simulink library "roblocks"  (Simulink 4.00)
values from neighbouring files (symbols this model uses):
  q = u(1:n)    [sldyn.m]
  qd = u(n+1:2*n)    [sldyn.m]
  qdd = accel(robot, u(1:n), u(n+1:2*n), u(2*n+1:3*n))    [sldyn.m]
undefined symbols (not defined in the file or in its folder): eul2tr, fkine, jacob0, jacobn, rne, robot, rpy2tr, tr2diff, tr2eul, tr2rpy, transl
libraries: simulink3 x2
settings Model: Creator=pic  LastModifiedBy=pic

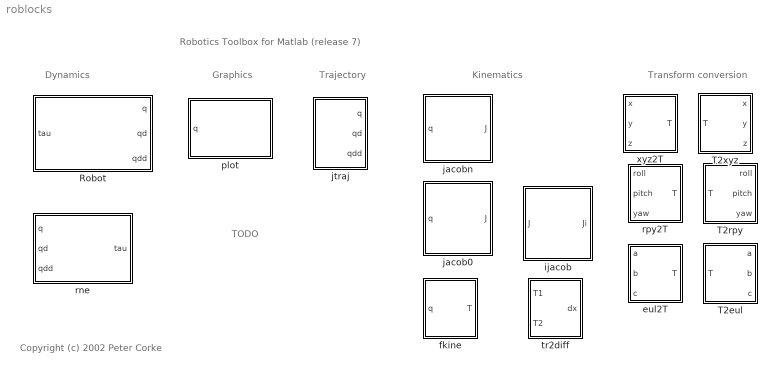
== system roblocks ==
  note: Robotics Toolbox for Matlab (release 7)
  note: TODO
  note: Copyright (c) 2002 Peter Corke
  note: Dynamics
  note: Graphics
  note: Kinematics
  note: Transform conversion
  note: Trajectory
  Robot : Subsystem  mask{robot=robot, q0=[0 0 0 0 0 0]}
      mask prompts: robot "Robot object"; q0 "Initial state"
      mask help: Rigid-body dynamic model of robot.
      mask init:
      | n = robot.n;
      | name = robot.name;
      settings: RTWFcnNameOpts=Auto  RTWFileNameOpts=Auto
      mask Help: Simulates the forward (direct) rigid-body dynamics of the robot described by the given robot object.
      mask Display:
      | port_label('input', 1, 'tau')
      | port_label('output', 1, 'q')
      | port_label('output', 2, 'qd')
      | port_label('output', 3, 'qdd')
      | text(0.1, 0.9,  robot.name, 'horizontalAlignment', 'left')
  T2eul : Subsystem
      settings: RTWFcnNameOpts=Auto  RTWFileNameOpts=Auto
      mask Description: Convert transform to Euler angles.
  T2rpy : Subsystem
      settings: RTWFcnNameOpts=Auto  RTWFileNameOpts=Auto
      mask Description: Convert transform to roll/pitch/yaw angles.
  T2xyz : Subsystem
      settings: RTWFcnNameOpts=Auto  RTWFileNameOpts=Auto
      mask Description: Convert transform to xyz scalars
  eul2T : Subsystem
      settings: RTWFcnNameOpts=Auto  RTWFileNameOpts=Auto
      mask Description: Convert Euler angles to transform.
  fkine : Subsystem  mask{robot=robot}
      mask prompts: robot "Robot object"
      mask help: Robot forward kinematics.
      settings: RTWFcnNameOpts=Auto  RTWFileNameOpts=Auto
      mask Help: Compute homogeneous transform for robot end-effector given joint angles.
      mask Display:
      | port_label('input', 1, 'q')
      | port_label('output', 1, 'T')
      | text(0.9, 0.9, robot.name,  'horizontalAlignment', 'right')
  ijacob : Subsystem
      settings: RTWFcnNameOpts=Auto  RTWFileNameOpts=Auto
      mask Description:
      | Robot inverse Jacobian for world coordinates.
      | 
      | Only valid for square jacobians (ie/ 6DOF robots)
      mask Display:
      | text(0.4, 0.7, 'J', 'verticalAlignment', 'top', 'horizontalAlignment', 'left')
      | text(0.65, 0.65, '-1', 'verticalAlignment', 'bottom', 'horizontalAlignment', 'right')
      | port_label('input', 1, 'J');
      | port_label('output', 1, 'Ji')
  "jacob0 " : Subsystem  mask{robot=robot}
      mask prompts: robot "Robot object"
      mask help: Robot Jacobian for end-effector coordinates
      mask init:
      | n=robot.n;
      settings: RTWFcnNameOpts=Auto  RTWFileNameOpts=Auto
      mask Display:
      | text(0.4, 0.7, 'J', 'verticalAlignment', 'top', 'horizontalAlignment', 'left')
      | text(0.4, 0.7, '0', 'verticalAlignment', 'bottom', 'horizontalAlignment', 'right')
      | text(0.5, 0.2, robot.name,  'horizontalAlignment', 'center')
      | port_label('input', 1, 'q')
      | port_label('output', 1, 'J')
  jacobn : Subsystem  mask{robot=robot}
      mask prompts: robot "Robot object"
      mask help: Robot Jacobian for end-effector coordinates
      mask init:
      | n=robot.n;
      settings: RTWFcnNameOpts=Auto  RTWFileNameOpts=Auto
      mask Display:
      | text(0.5, 0.4, 'J', 'verticalAlignment', 'top', 'horizontalAlignment', 'left')
      | text(0.5, 0.4, 'n', 'verticalAlignment', 'bottom', 'horizontalAlignment', 'right')
      | text(0.9, 0.9, robot.name,  'horizontalAlignment', 'right')
      | port_label('input', 1, 'q')
      | port_label('output', 1, 'J')
  jtraj : Subsystem  mask{q0=[0 0 0 0 0 0], qf=[pi/4 pi/2 -pi/2 0 0 0], tmax=10}
      mask help: Joint interpolated trajectory.
      mask init:
      | n = length(q0);
      | if length(q0) ~= length(qf) ,
      |  error('q0 and qf must be same length')
      | end
      | t=[0:100]'/100*tmax;
      | [q,qd,qdd] = jtraj(q0, qf, t);
      settings: RTWFcnNameOpts=Auto  RTWFileNameOpts=Auto
      mask Help:
      | Generate quintic polynomial to move from initial to final joint angles as specified.  Initial and final velocity are assumed to be zero.
      | 
      | Outputs joint angles as well as joint angle rates.
      mask Display:
      | port_label('output', 1, 'q')
      | port_label('output', 2, 'qd')
      | port_label('output', 3, 'qdd')
  plot : Subsystem  mask{robot=robot}
      mask prompts: robot "Name of robot"
      mask help: Graphical robot display.
      mask init:
      | plot(robot,zeros(1,robot.n))
      settings: RTWFcnNameOpts=Auto  RTWFileNameOpts=Auto
      mask Help: This block graphically displays the named robot
      mask Display: text(0.5, 0.5,  robot.name, 'horizontalAlignment', 'center')
  rne : Subsystem  mask{robot=robot, grav=[0 0 9.81]}
      mask prompts: robot "Robot object"; grav "Gravity"
      mask help: Rigid-body inverse dynamics.
      mask init:
      | n=robot.n;
      settings: RTWFcnNameOpts=Auto  RTWFileNameOpts=Auto
      mask Help: Given a robot dynamic model and joint angle, rate and acceleration determine the required joint torque.  Useful for computed and inverse torque control schemes.
      mask Display:
      | port_label('output', 1, 'tau')
      | port_label('input', 1, 'q')
      | port_label('input', 2, 'qd')
      | port_label('input', 3, 'qdd')
      | text(0.9, 0.9,  robot.name, 'horizontalAlignment', 'right')
  rpy2T : Subsystem
      settings: RTWFcnNameOpts=Auto  RTWFileNameOpts=Auto
      mask Description: Convert roll/pitch/yaw angles to transform.
  tr2diff : Subsystem  mask{robot=robot}
      mask prompts: robot "Robot object"
      mask help: Robot forward kinematics.
      settings: RTWFcnNameOpts=Auto  RTWFileNameOpts=Auto
      mask Help: Compute homogeneous transform for robot end-effector given joint angles.
      mask Display:
      | port_label('input', 1, 'T1')
      | port_label('input', 2, 'T2')
      | port_label('output', 1, 'dx')
  xyz2T : Subsystem
      settings: RTWFcnNameOpts=Auto  RTWFileNameOpts=Auto
      mask Description: Convert xyz scalars to transform.

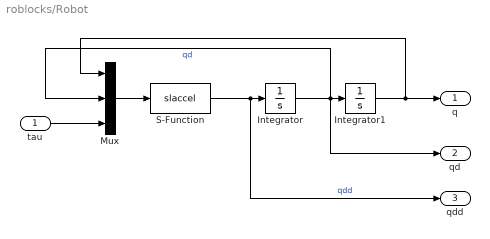
== system roblocks/Robot ==
  tau : Inport  Port=1
  Integrator : Integrator  ExternalReset=none  InitialConditionSource=internal  InitialCondition=0  LimitOutput=off  UpperSaturationLimit=inf  LowerSaturationLimit=-inf  ShowSaturationPort=off  ShowStatePort=off  AbsoluteTolerance=auto
  Integrator1 : Integrator  ExternalReset=none  InitialConditionSource=internal  InitialCondition=0  LimitOutput=off  UpperSaturationLimit=inf  LowerSaturationLimit=-inf  ShowSaturationPort=off  ShowStatePort=off  AbsoluteTolerance=auto
  Mux : Mux  Inputs=3
  S-Function : S-Function  FunctionName=slaccel  Parameters=robot  PortCounts=[]  SFunctionModules=''
  q : Outport  Port=1
  qd : Outport  Port=2
  qdd : Outport  Port=3
  wires:
  S-Function/1 -> qdd/1, Integrator/1  "qdd"
  Mux/1 -> S-Function/1
  Integrator/1 -> qd/1, Integrator1/1, Mux/2  "qd"
  tau/1 -> Mux/3
  Integrator1/1 -> q/1, Mux/1

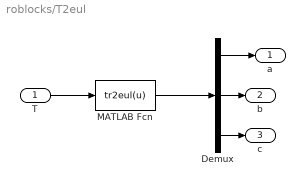
== system roblocks/T2eul ==
  T : Inport  Port=1
  Demux : Demux  Outputs=3  BusSelectionMode=off
  MATLAB Fcn : MATLABFcn  MATLABFcn=tr2eul(u)  OutputDimensions=3  OutputSignalType=auto  Output1D=on
  a : Outport  Port=1
  b : Outport  Port=2
  c : Outport  Port=3
  wires:
  Demux/3 -> c/1
  Demux/2 -> b/1
  Demux/1 -> a/1
  MATLAB Fcn/1 -> Demux/1
  T/1 -> MATLAB Fcn/1

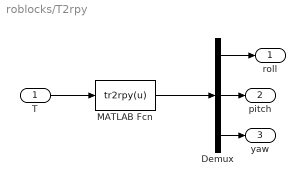
== system roblocks/T2rpy ==
  T : Inport  Port=1
  Demux : Demux  Outputs=3  BusSelectionMode=off
  MATLAB Fcn : MATLABFcn  MATLABFcn=tr2rpy(u)  OutputDimensions=3  OutputSignalType=auto  Output1D=on
  roll : Outport  Port=1
  pitch : Outport  Port=2
  yaw : Outport  Port=3
  wires:
  Demux/3 -> yaw/1
  Demux/2 -> pitch/1
  Demux/1 -> roll/1
  MATLAB Fcn/1 -> Demux/1
  T/1 -> MATLAB Fcn/1

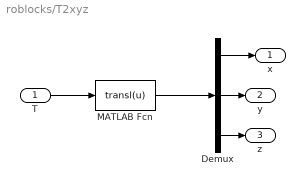
== system roblocks/T2xyz ==
  T : Inport  Port=1
  Demux : Demux  Outputs=3  BusSelectionMode=off
  MATLAB Fcn : MATLABFcn  MATLABFcn=transl(u)  OutputDimensions=3  OutputSignalType=auto  Output1D=on
  x : Outport  Port=1
  y : Outport  Port=2
  z : Outport  Port=3
  wires:
  T/1 -> MATLAB Fcn/1
  MATLAB Fcn/1 -> Demux/1
  Demux/1 -> x/1
  Demux/2 -> y/1
  Demux/3 -> z/1

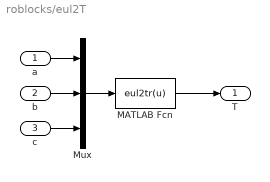
== system roblocks/eul2T ==
  a : Inport  Port=1
  b : Inport  Port=2
  c : Inport  Port=3
  MATLAB Fcn : MATLABFcn  MATLABFcn=eul2tr(u)  OutputDimensions=[4 4]  OutputSignalType=auto  Output1D=off
  Mux : Mux  Inputs=3
  T : Outport  Port=1
  wires:
  c/1 -> Mux/3
  MATLAB Fcn/1 -> T/1
  Mux/1 -> MATLAB Fcn/1
  a/1 -> Mux/1
  b/1 -> Mux/2

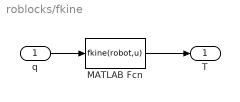
== system roblocks/fkine ==
  q : Inport  Port=1
  MATLAB Fcn : MATLABFcn  MATLABFcn=fkine(robot,u)  OutputDimensions=[4 4]  OutputSignalType=auto  Output1D=off
  T : Outport  Port=1
  wires:
  q/1 -> MATLAB Fcn/1
  MATLAB Fcn/1 -> T/1

== system roblocks/ijacob ==
  J : Inport  Port=1
  inverse jacobian : MATLABFcn  MATLABFcn=inv(u)  OutputDimensions=-1  OutputSignalType=auto  Output1D=off
  Ji : Outport  Port=1
  wires:
  inverse jacobian/1 -> Ji/1
  J/1 -> inverse jacobian/1

== system roblocks/jacob0  ==
  q : Inport  Port=1
  MATLAB Fcn : MATLABFcn  MATLABFcn=jacob0(robot,u)  OutputDimensions=[6 n]  OutputSignalType=auto  Output1D=off
  J : Outport  Port=1
  wires:
  MATLAB Fcn/1 -> J/1
  q/1 -> MATLAB Fcn/1

== system roblocks/jacobn ==
  q : Inport  Port=1
  MATLAB Fcn : MATLABFcn  MATLABFcn=jacobn(robot,u)  OutputDimensions=[6 n]  OutputSignalType=auto  Output1D=off
  J : Outport  Port=1
  wires:
  MATLAB Fcn/1 -> J/1
  q/1 -> MATLAB Fcn/1

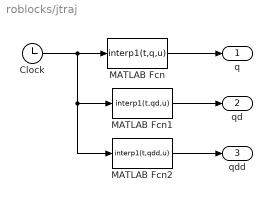
== system roblocks/jtraj ==
  Clock : Clock
      settings: DisplayTime=off  Decimation=10
  MATLAB Fcn : MATLABFcn  MATLABFcn=interp1(t,q,u)  OutputDimensions=n  OutputSignalType=auto  Output1D=on
  MATLAB Fcn1 : MATLABFcn  MATLABFcn=interp1(t,qd,u)  OutputDimensions=n  OutputSignalType=auto  Output1D=on
  MATLAB Fcn2 : MATLABFcn  MATLABFcn=interp1(t,qdd,u)  OutputDimensions=n  OutputSignalType=auto  Output1D=on
  q : Outport  Port=1
  qd : Outport  Port=2
  qdd : Outport  Port=3
  wires:
  MATLAB Fcn/1 -> q/1
  MATLAB Fcn1/1 -> qd/1
  Clock/1 -> MATLAB Fcn/1, MATLAB Fcn1/1, MATLAB Fcn2/1
  MATLAB Fcn2/1 -> qdd/1

== system roblocks/plot ==
  q : Inport  Port=1
  S-Function : S-Function  FunctionName=slplotbot  Parameters=robot  PortCounts=[]  SFunctionModules=''
  wires:
  q/1 -> S-Function/1

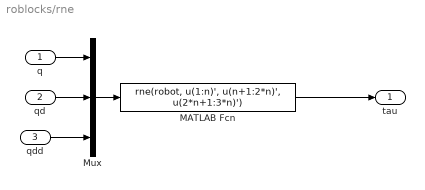
== system roblocks/rne ==
  q : Inport  Port=1
  qd : Inport  Port=2
  qdd : Inport  Port=3
  MATLAB Fcn : MATLABFcn  MATLABFcn=rne(robot, u(1:n)', u(n+1:2*n)', u(2*n+1:3*n)')  OutputDimensions=n  OutputSignalType=auto  Output1D=on
  Mux : Mux  Inputs=3
  tau : Outport  Port=1
  wires:
  Mux/1 -> MATLAB Fcn/1
  q/1 -> Mux/1
  qd/1 -> Mux/2
  qdd/1 -> Mux/3
  MATLAB Fcn/1 -> tau/1

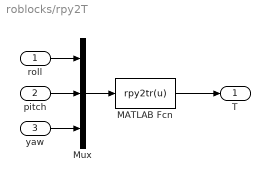
== system roblocks/rpy2T ==
  roll : Inport  Port=1
  pitch : Inport  Port=2
  yaw : Inport  Port=3
  MATLAB Fcn : MATLABFcn  MATLABFcn=rpy2tr(u)  OutputDimensions=[4 4]  OutputSignalType=auto  Output1D=off
  Mux : Mux  Inputs=3
  T : Outport  Port=1
  wires:
  yaw/1 -> Mux/3
  MATLAB Fcn/1 -> T/1
  Mux/1 -> MATLAB Fcn/1
  roll/1 -> Mux/1
  pitch/1 -> Mux/2

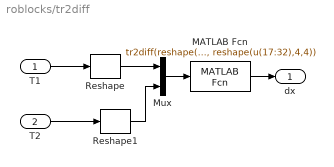
== system roblocks/tr2diff ==
  T1 : Inport  Port=1
  T2 : Inport  Port=2
  MATLAB Fcn : MATLABFcn  MATLABFcn=tr2diff(reshape(u(1:16),4,4), reshape(u(17:32),4,4))  OutputDimensions=6  OutputSignalType=auto  Output1D=on
  Mux : Mux  Inputs=2
  Reshape : simulink3/Signals & Systems/Reshape  OutputDimensionality=1-D array  OutputDimensions=[1,1]
  Reshape1 : simulink3/Signals & Systems/Reshape  OutputDimensionality=1-D array  OutputDimensions=[1,1]
  dx : Outport  Port=1
  wires:
  MATLAB Fcn/1 -> dx/1
  T1/1 -> Reshape/1
  T2/1 -> Reshape1/1
  Mux/1 -> MATLAB Fcn/1
  Reshape/1 -> Mux/1
  Reshape1/1 -> Mux/2

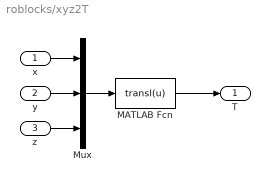
== system roblocks/xyz2T ==
  x : Inport  Port=1
  y : Inport  Port=2
  z : Inport  Port=3
  MATLAB Fcn : MATLABFcn  MATLABFcn=transl(u)  OutputDimensions=[4 4]  OutputSignalType=auto  Output1D=off
  Mux : Mux  Inputs=3
  T : Outport  Port=1
  wires:
  y/1 -> Mux/2
  x/1 -> Mux/1
  Mux/1 -> MATLAB Fcn/1
  MATLAB Fcn/1 -> T/1
  z/1 -> Mux/3
